simulink model "transferfunction12B_Pcontrol"  (R2022b)
settings: Solver=VariableStepAuto  StartTime=t(1)  StopTime=t(end)  FixedStep=t(2)-t(1)  MaxStep=Auto  MinStep=Auto  RelTol=1e-3
values from neighbouring files (symbols this model uses):
  EX3_SENS_DEN = [1]    [Analysis.m]
  EX3_SENS_NUM = [1]    [Analysis.m]
  K = 50000    [Analysis.m]
settings Model: Creator=u0062516  LastModifiedBy=debber
settings SolverCC: InitialStep=Auto
settings DataIOCC: ExternalInput=[t, x]  LoadExternalInput=on  SaveFormat=Array  SignalLogging=off  DSMLogging=off  OutputSaveName=y
settings HardwareCC: TargetBitPerLong=64  TargetBitPerPointer=64  TargetBitPerSizeT=64  TargetBitPerPtrDiffT=64  TargetLongLongMode=on  TargetIntDivRoundTo=Zero  TargetEndianess=LittleEndian  TargetWordSize=64  TargetHWDeviceType=MATLAB Host  ProdEqTarget=off
settings RTWCC: Description=Rapid Simulation Target  SystemTargetFile=rsim.tlc  TemplateMakefile=rsim_default_tmf
settings RSimTargetCC: TargetLangStandard=C99 (ISO)  OptimizeReductions=off

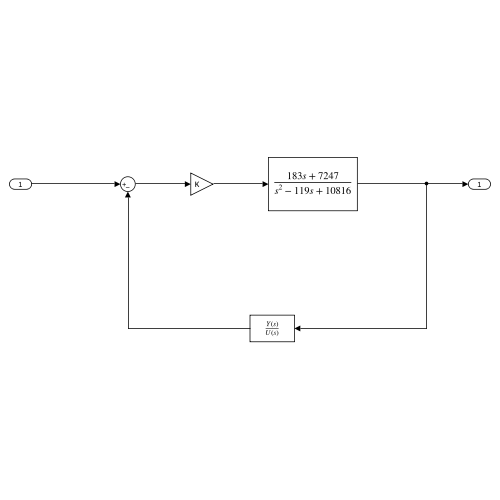
[thumbnail: Simulink's stored preview of the top-level diagram]
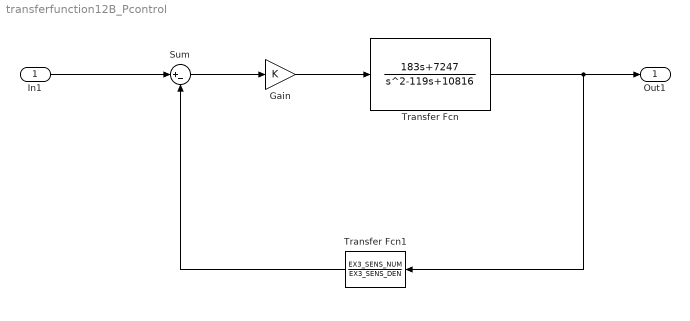
== system transferfunction12B_Pcontrol ==
  In1 : Inport
  Gain : Gain  Gain=K
  Sum : Sum  Inputs=|+-
  Transfer Fcn : TransferFcn  Numerator=[183 7247]  Denominator=[1 -119 10816]  ParameterTunability=Unconstrained
  Transfer Fcn1 : TransferFcn  Numerator=EX3_SENS_NUM  Denominator=EX3_SENS_DEN
  Out1 : Outport
  wires:
  Gain/1 -> Transfer Fcn/1
  In1/1 -> Sum/1
  Sum/1 -> Gain/1
  Transfer Fcn/1 -> Out1/1, Transfer Fcn1/1
  Transfer Fcn1/1 -> Sum/2
